simulink model "Final_Simulink_Model_assignment_2"  (R2022b)
settings: Solver=FixedStepAuto  StartTime=0.0  StopTime=inf  FixedStep=1e-3  RelTol=1e-3  EnableMultiTasking=on
undefined symbols (not defined in the file): A0, A1, ATR_PULSE_WIDTH, ATR_PUSLE_WIDTH, D0, D1, D10, D11, D12, D13, D2, D3, D4, D5, D6, D7, D8, D9, LRL, magnitude, PTA0, PTA1, PTA2, PTB2, PTB23, PTB3, PTB9, PTC16, PTC17, PTC2, PTC3, PTC4, PTD0, PTD1, PTD2, PTD3, REF_PERIOD, REF_PREIOD, VENT_PULSE_WIDTH
libraries: frdmk64flib x30, etargetslib x9, dspstat3 x1
(part 1 of 2)
settings Model: ExtModeTrigDuration=5  Creator=clara  LastModifiedBy=dinghao
settings OptimizationCC: EnhancedBackFolding=on  PassReuseOutputArgsAs=Individual arguments  ZeroExternalMemoryAtStartup=off  ZeroInternalMemoryAtStartup=off  MaxStackSize=64  OptimizeBlockOrder=speed  DifferentSizesBufferReuse=on  OptimizationCustomize=off  EfficientTunableParamExpr=on
settings DebuggingCC: ParameterTunabilityLossMsg=error
settings HardwareCC: ProdBitPerPointer=32  ProdBitPerSizeT=32  ProdBitPerPtrDiffT=32  ProdLargestAtomicInteger=Long  ProdLargestAtomicFloat=Double  ProdWordSize=32  ProdHWDeviceType=ARM Compatible->ARM Cortex
settings ModelReferenceCC: EnableRefExpFcnMdlSchedulingChecks=on
settings SFSimCC: MATLABDynamicMemAlloc=off
settings RTWCC: Description=Embedded Coder  SystemTargetFile=ert.tlc  HardwareBoard=NXP FRDM-K64F  TLCOptions="-aInlineSetEventsForThisBaseRateFcn=TLC_FALSE -aSuppressMultiTaskScheduler=TLC_FALSE  -aRateBasedStepFcn=0"  TemplateMakefile=ert_default_tmf  Toolchain=GNU Tools for ARM Embedded Processors
settings CodeAppCC: ForceParamTrailComments=on  IgnoreCustomStorageClasses=off  OperatorAnnotations=on  SimulinkDataObjDesc=on  SFDataObjDesc=on  InsertBlockDesc=on
settings ERTTargetCC: ExtModeTransport=4  ExtModeMexFile=sendToCommService

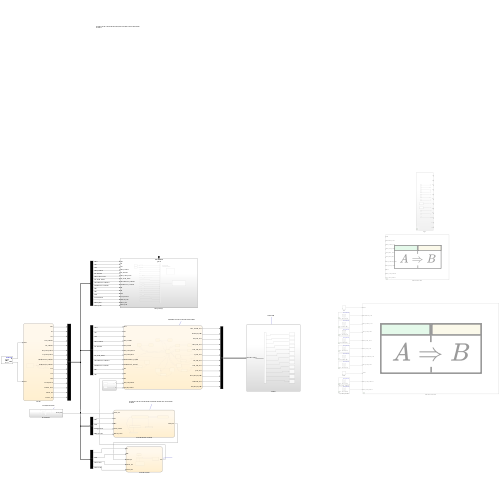
[thumbnail: Simulink's stored preview of the top-level diagram]
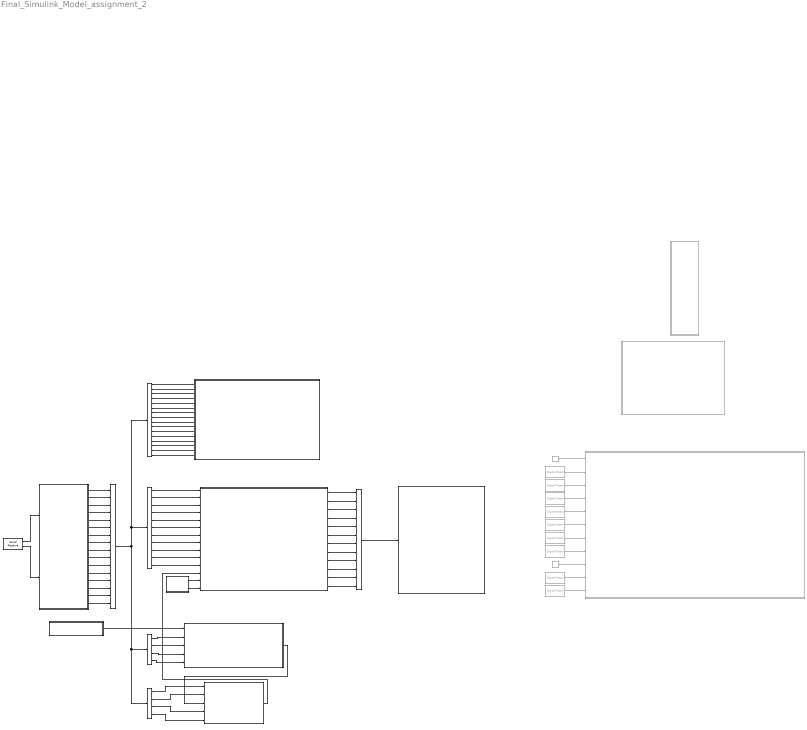
== system Final_Simulink_Model_assignment_2 ==
  note: the model is used to find the desired pacing rate with response factor under different conditions
  note: Find target activity level
  note: Slowly or linearly increase the current heart rate to the desired value
  note: the model is used to find the desired pacing rate with response factor under different conditions
  note: Output hiding
  note: Eight different modes with and without rate adaptive
  ATR_CMP_DETECT : frdmk64flib/Digital Read  Commented=on  Whichpin=PTC16 (D0)  SampleTime=-1
  Accelerometer1 : Subsystem
  Bus Creator : BusCreator  Inputs=16
  Bus Creator1 : BusCreator  Inputs=12
  Bus Selector : BusSelector  OutputSignals=mode,LRL,URL,VENT_Amplitude,ATR_Amplitude,VENT_PULSE_WIDTH,ATR_PULSE_WIDTH,VENTSENSITIVITY_Amplitude,ATRSENSITIVITY_Amplitude,ARP,VRP
  Bus Selector1 : BusSelector  OutputSignals=mode,LRL,URL,VENT_Amplitude,ATR_Amplitude,VENT_PULSE_WIDTH,ATR_PULSE_WIDTH,VENTSENSITIVITY_Amplitude,ATRSENSITIVITY_Amplitude,ARP,VRP,MSR,Activity_threshold,Response_Factor,Reaction_time,Recovery_time
  Bus Selector2 : BusSelector  OutputSignals=LRL,MSR,Activity_threshold,Response_Factor
  Bus Selector3 : BusSelector  OutputSignals=LRL,MSR,Reaction_time,Recovery_time
  COM_IN1 : Stateflow chart  TreatAsAtomicUnit=on
  Chart1 : Stateflow chart  TreatAsAtomicUnit=on
      settings: PortSchema="{\"entries\":[{\"content\":{\"sides\":[{\"content\":{\"connectorIds\":[\"In8\",\"In1\",\"In6\",\"In2\",\"In3\",\"In4\",\"In5\",\"In7\",\"In9\",\"In10\",\"In11\",\"In12\",\"In13\",\"In14\"]},\"type\":\"ConnectorPlacement.EquallySpacedRectSide\",\"uuid\":\"411cfc43-89c3-4653-9fab-0da98be593d3\"},{\"content\":{\"connectorIds\":[\"Out1\",\"Out2\",\"Out3\",\"Out4\",\"Out5\",\"Out6\",\"Out7\",\"Out8\",\"Out9\",\"Out10\",\"Out11\",\"Out12\"],\"side\":\"RIGHT\"},\"type\":\"ConnectorPlacement.EquallySpacedRectSide\",\"uuid\":\"ad1683f7-26aa-4767-b656-f3b731cb8235\"},{\"content\":{\"connectorIds\":[],\"side\":\"TOP\"},\"type\":\"ConnectorPlacement.EquallySpacedRectSide\",\"uuid\":\"fbccba07-c1cc-4c9f-8e56-0bdfb6912bb8\"}]},\"type\":\"ConnectorPlacement.EquallySpacedConnector\",\"uuid\":\"0c618a7f-9484-4de3-a6ac-3c8308721375\"}],\"packageUris\":[\"http://schema.mathworks.com/mf0/Connector/R2020b\"],\"version\":\"1.0\"}"
  Digital Read : frdmk64flib/Digital Read  Commented=on  Whichpin=PTB9 (D2)  SampleTime=-1
  Digital Read1 : frdmk64flib/Digital Read  Commented=on  Whichpin=PTD0 (D10)  SampleTime=-1
  Digital Read2 : frdmk64flib/Digital Read  Commented=on  Whichpin=PTD2 (D11)  SampleTime=-1
  Digital Read3 : frdmk64flib/Digital Read  Commented=on  Whichpin=PTA0 (D8)  SampleTime=-1
  Digital Read4 : frdmk64flib/Digital Read  Commented=on  Whichpin=PTD3 (D12)  SampleTime=-1
  Digital Read5 : frdmk64flib/Digital Read  Commented=on  Whichpin=PTC4 (D9)  SampleTime=-1
  Digital Read6 : frdmk64flib/Digital Read  Commented=on  Whichpin=PTD1 (D13)  SampleTime=-1
  Find the desired rate for pacing1 : Stateflow chart  TreatAsAtomicUnit=on
  Find the pacing rate1 : Stateflow chart  TreatAsAtomicUnit=on
  INPUT 1 : Subsystem  Commented=on
  Mode : Constant  Commented=on
  OUTPUT1 : Subsystem
  Requirements Table : Requirements Table  Commented=on  TreatAsAtomicUnit=on
  Requirements Table1 : Requirements Table  Commented=on  TreatAsAtomicUnit=on
  Serial Receive1 : frdmk64flib/Serial Receive  SCIModule=0  Baudrate=uint32(9600)  Parity=None  StopBits=1  HardwareFlowControl=None  ByteOrder=LittleEndian  DataType=uint8  DataLength=35  BlockingMode=off  OutputStatus=on  SampleTime=-1
  State : Constant  Commented=on
  Subsystem1 : Subsystem
  VENT_CMP_DETECT : frdmk64flib/Digital Read  Commented=on  Whichpin=PTC17 (D1)  SampleTime=-1
  send_params()1 : Subsystem
  wires:
  Accelerometer1/1(Activity_level) -> Find the desired rate for pacing1/1(Activity_level)
  Subsystem1/2(Out8) -> Chart1/14(ATR_CMP_DETECT)
  Serial Receive1/2 -> COM_IN1/2(status)
  Subsystem1/1(Out7) -> Chart1/13(VENT_CMP_DETECT)
  Find the pacing rate1/1(rate) -> Chart1/12(Rate)
  Find the desired rate for pacing1/1(Desired_rate) -> Find the pacing rate1/3(Desired_rate)
  Serial Receive1/1 -> COM_IN1/1(rxdata)
  COM_IN1/1(mode) -> Bus Creator/1
  COM_IN1/2(LRL) -> Bus Creator/2
  COM_IN1/3(URL) -> Bus Creator/3
  COM_IN1/4(VENT_Amplitude) -> Bus Creator/4
  COM_IN1/5(ATR_Amplitude) -> Bus Creator/5
  COM_IN1/6(VENT_PULSE_WIDTH) -> Bus Creator/6
  COM_IN1/7(ATR_PULSE_WIDTH) -> Bus Creator/7
  COM_IN1/8(VENTSENSITIVITY_Amplitude) -> Bus Creator/8
  COM_IN1/9(ATRSENSITIVITY_Amplitude) -> Bus Creator/9
  COM_IN1/10(ARP) -> Bus Creator/10
  COM_IN1/11(VRP) -> Bus Creator/11
  COM_IN1/12(MSR) -> Bus Creator/12
  COM_IN1/13(Activity_threshold) -> Bus Creator/13
  COM_IN1/14(Response_Factor) -> Bus Creator/14
  COM_IN1/15(Reaction_time) -> Bus Creator/15
  COM_IN1/16(Recovery_time) -> Bus Creator/16
  Bus Creator/1 -> Bus Selector3/1, Bus Selector2/1, Bus Selector1/1, Bus Selector/1
  Bus Selector/1 -> Chart1/8(mode)  "<mode>"
  Bus Selector/4 -> Chart1/2(VENT_Amplitude)  "<VENT_Amplitude>"
  Bus Selector/5 -> Chart1/3(ATR_Amplitude)  "<ATR_Amplitude>"
  Bus Selector/6 -> Chart1/4(VENT_PULSE_WIDTH)  "<VENT_PULSE_WIDTH>"
  Bus Selector/7 -> Chart1/5(ATR_PULSE_WIDTH)  "<ATR_PULSE_WIDTH>"
  Bus Selector/8 -> Chart1/7(VENTSENSITIVITY_Amplitude)  "<VENTSENSITIVITY_Amplitude>"
  Bus Selector/9 -> Chart1/9(ATRSENSITIVITY_Amplitude)  "<ATRSENSITIVITY_Amplitude>"
  Bus Selector/10 -> Chart1/10(ARP)  "<ARP>"
  Bus Selector/11 -> Chart1/11(VRP)  "<VRP>"
  Bus Selector/2 -> Chart1/1(LRL)  "<LRL>"
  Bus Selector/3 -> Chart1/6(URL)  "<URL>"
  Bus Selector1/1 -> send_params()1/1(mode)  "<mode>"
  Bus Selector1/2 -> send_params()1/2(LRL)  "<LRL>"
  Bus Selector1/3 -> send_params()1/3(URL)  "<URL>"
  Bus Selector1/4 -> send_params()1/4(VENT_Amplitude)  "<VENT_Amplitude>"
  Bus Selector1/5 -> send_params()1/5(ATR_Amplitude)  "<ATR_Amplitude>"
  Bus Selector1/6 -> send_params()1/6(VENT_PULSE_WIDTH)  "<VENT_PULSE_WIDTH>"
  Bus Selector1/7 -> send_params()1/7(ATR_PULSE_WIDTH)  "<ATR_PULSE_WIDTH>"
  Bus Selector1/8 -> send_params()1/8(VENTSENSITIVITY_Amplitude)  "<VENTSENSITIVITY_Amplitude>"
  Bus Selector1/9 -> send_params()1/9(ATRSENSITIVITY_Amplitude)  "<ATRSENSITIVITY_Amplitude>"
  Bus Selector1/10 -> send_params()1/10(ARP)  "<ARP>"
  Bus Selector1/11 -> send_params()1/11(VRP)  "<VRP>"
  Bus Selector1/12 -> send_params()1/12(MSR)  "<MSR>"
  Bus Selector1/13 -> send_params()1/13(Activity_threshold)  "<Activity_threshold>"
  Bus Selector1/14 -> send_params()1/14(Response_Factor)  "<Response_Factor>"
  Bus Selector1/15 -> send_params()1/15(Reaction_time)  "<Reaction_time>"
  Bus Selector1/16 -> send_params()1/16(Recovery_time)  "<Recovery_time>"
  Bus Selector2/1 -> Find the desired rate for pacing1/2(LRL)  "<LRL>"
  Bus Selector2/2 -> Find the desired rate for pacing1/3(MSR)  "<MSR>"
  Bus Selector2/3 -> Find the desired rate for pacing1/4(Activity_threshold)  "<Activity_threshold>"
  Bus Selector2/4 -> Find the desired rate for pacing1/5(Response_Factor)  "<Response_Factor>"
  Bus Selector3/1 -> Find the pacing rate1/1(LRL)  "<LRL>"
  Bus Selector3/2 -> Find the pacing rate1/2(MSR)  "<MSR>"
  Bus Selector3/3 -> Find the pacing rate1/4(Reaction_time)  "<Reaction_time>"
  Bus Selector3/4 -> Find the pacing rate1/5(Recovery_time)  "<Recovery_time>"
  Chart1/1(PACE_CHARGE_CTRL) -> Bus Creator1/1
  Chart1/2(PACING_REF_PWM) -> Bus Creator1/2
  Chart1/3(ATR_PACE_CTRL) -> Bus Creator1/3
  Chart1/4(VENT_PACE_CTRL) -> Bus Creator1/4
  Chart1/5(PACE_GND_CTRL) -> Bus Creator1/5
  Chart1/6(Z_VENT_CTRL) -> Bus Creator1/6
  Chart1/7(ATR_GND_CTRL) -> Bus Creator1/7
  Chart1/8(VENT_GND_CTRL) -> Bus Creator1/8
  Chart1/9(Z_ATR_CTRL) -> Bus Creator1/9
  Chart1/10(VENT_CMP_REF_PWM) -> Bus Creator1/10
  Chart1/11(FRONTEND_CTRL) -> Bus Creator1/11
  Chart1/12(ATR_CMP_REF_PWM) -> Bus Creator1/12
  Bus Creator1/1 -> OUTPUT1/1(CONTROL OUTPUT)
  State/1 -> Requirements Table1/1(State)
  Digital Read/1 -> Requirements Table1/7(PACE_CHARGE_CTRL)
  Digital Read2/1 -> Requirements Table1/6(ATR_GND_CTRL)
  Digital Read5/1 -> Requirements Table1/3(VENT_PACE_CTRL)
  Digital Read6/1 -> Requirements Table1/2(FRONTEND_CTRL)
  ATR_CMP_DETECT/1 -> Requirements Table1/11(ATR_CMP_DETECT)
  Digital Read4/1 -> Requirements Table1/4(VENT_GND_CTRL)
  VENT_CMP_DETECT/1 -> Requirements Table1/10(VENT_CMP_DETECT)
  Digital Read3/1 -> Requirements Table1/5(ATR_PACE_CTRL)
  Mode/1 -> Requirements Table1/9(Mode)
  Digital Read1/1 -> Requirements Table1/8(PACE_GND_CTRL)

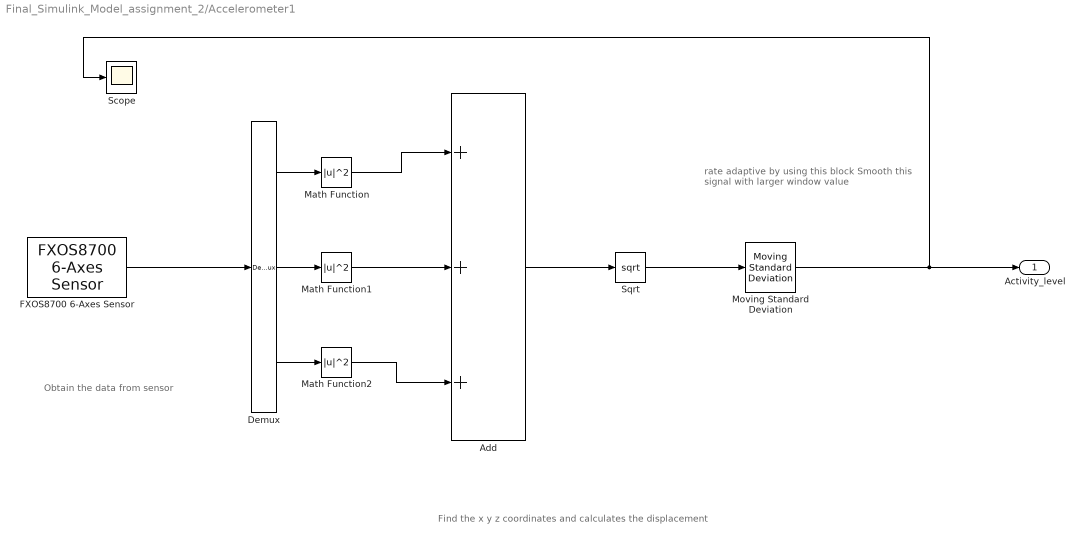
== system Final_Simulink_Model_assignment_2/Accelerometer1 ==
  note: Obtain the data from sensor
  note: Find the x y z coordinates and calculates the displacement
  note: rate adaptive by using this block
      | Smooth this signal with larger window value
  Add : Sum  Inputs=+++  OutDataTypeStr=double
  Demux : Demux  Outputs=3
  FXOS8700 6-Axes Sensor : frdmk64flib/FXOS8700 6-Axes Sensor  Activesensor=Accelerometer only  ODR=800Hz  HybridODR=400Hz  Accelfullrange=-4g to +4g  SampleTime=0.01
  Math Function : Math  Operator=magnitude^2  OutDataTypeStr=double
  Math Function1 : Math  Operator=magnitude^2  OutDataTypeStr=double
  Math Function2 : Math  Operator=magnitude^2  OutDataTypeStr=double
  Moving Standard Deviation : dspstat3/Moving Standard Deviation  Method=Sliding window  ForgettingFactorPort=off  SpecifyWindowLength=on  WindowLength=400  OverlapLength=399  AllowArbitraryInputLength=off  ForgettingFactor=0.9  SimulateUsing=Code generation
  Scope : Scope
  Sqrt : Sqrt  OutDataTypeStr=double
  Activity_level : Outport  OutDataTypeStr=double
  wires:
  FXOS8700 6-Axes Sensor/1 -> Demux/1
  Demux/1 -> Math Function/1
  Demux/2 -> Math Function1/1
  Demux/3 -> Math Function2/1
  Math Function/1 -> Add/1
  Math Function2/1 -> Add/3
  Math Function1/1 -> Add/2
  Add/1 -> Sqrt/1
  Sqrt/1 -> Moving Standard Deviation/1
  Moving Standard Deviation/1 -> Scope/1, Activity_level/1

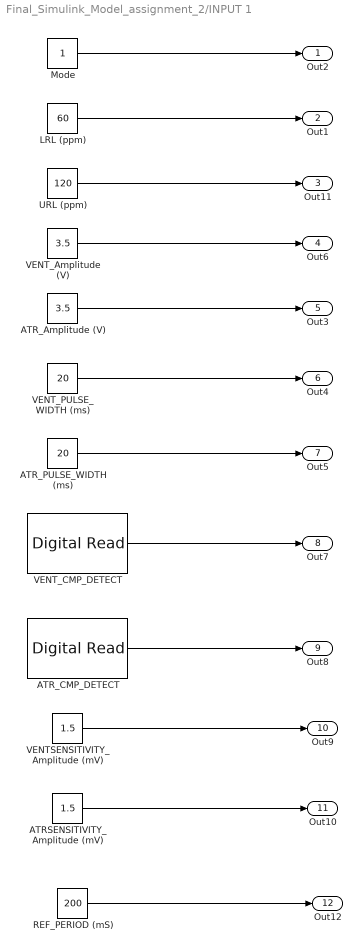
== system Final_Simulink_Model_assignment_2/INPUT 1 ==
  ATRSENSITIVITY_Amplitude (mV) : Constant  Value=1.5
  ATR_Amplitude (V) : Constant  Value=3.5
  ATR_CMP_DETECT : frdmk64flib/Digital Read  Whichpin=PTC16 (D0)  SampleTime=-1
  ATR_PULSE_WIDTH (ms) : Constant  Value=20
  LRL (ppm) : Constant  Value=60
  Mode : Constant
  REF_PERIOD (mS) : Constant  Value=200
  URL (ppm) : Constant  Value=120
  VENTSENSITIVITY_Amplitude (mV) : Constant  Value=1.5
  VENT_Amplitude (V) : Constant  Value=3.5
  VENT_CMP_DETECT : frdmk64flib/Digital Read  Whichpin=PTC17 (D1)  SampleTime=-1
  VENT_PULSE_WIDTH (ms) : Constant  Value=20
  Out2 : Outport
  Out1 : Outport  Port=2
  Out11 : Outport  Port=3
  Out6 : Outport  Port=4
  Out3 : Outport  Port=5
  Out4 : Outport  Port=6
  Out5 : Outport  Port=7
  Out7 : Outport  Port=8
  Out8 : Outport  Port=9
  Out9 : Outport  Port=10
  Out10 : Outport  Port=11
  Out12 : Outport  Port=12
  wires:
  LRL (ppm)/1 -> Out1/1
  VENT_PULSE_WIDTH (ms)/1 -> Out4/1
  VENT_Amplitude (V)/1 -> Out6/1
  URL (ppm)/1 -> Out11/1
  Mode/1 -> Out2/1
  ATR_Amplitude (V)/1 -> Out3/1
  ATR_PULSE_WIDTH (ms)/1 -> Out5/1
  VENT_CMP_DETECT/1 -> Out7/1
  ATR_CMP_DETECT/1 -> Out8/1
  VENTSENSITIVITY_Amplitude (mV)/1 -> Out9/1
  ATRSENSITIVITY_Amplitude (mV)/1 -> Out10/1
  REF_PERIOD (mS)/1 -> Out12/1

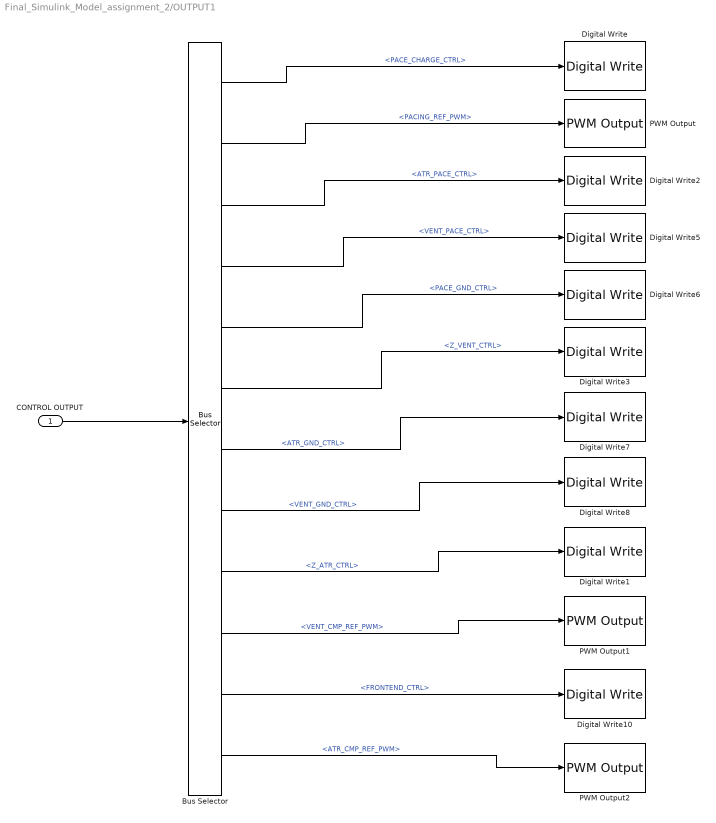
== system Final_Simulink_Model_assignment_2/OUTPUT1 ==
  CONTROL OUTPUT : Inport
  Bus Selector : BusSelector  OutputSignals=PACE_CHARGE_CTRL,PACING_REF_PWM,ATR_PACE_CTRL,VENT_PACE_CTRL,PACE_GND_CTRL,Z_VENT_CTRL,ATR_GND_CTRL,VENT_GND_CTRL,Z_ATR_CTRL,VENT_CMP_REF_PWM,FRONTEND_CTRL,ATR_CMP_REF_PWM
  Digital Write : frdmk64flib/Digital Write  Whichpin=PTB9 (D2)
  Digital Write1 : frdmk64flib/Digital Write  Whichpin=PTB23 (D4)
  Digital Write10 : frdmk64flib/Digital Write  Whichpin=PTD1 (D13)
  Digital Write2 : frdmk64flib/Digital Write  Whichpin=PTA0 (D8)
  Digital Write3 : frdmk64flib/Digital Write  Whichpin=PTC3 (D7)
  Digital Write5 : frdmk64flib/Digital Write  Whichpin=PTC4 (D9)
  Digital Write6 : frdmk64flib/Digital Write  Whichpin=PTD0 (D10)
  Digital Write7 : frdmk64flib/Digital Write  Whichpin=PTD2 (D11)
  Digital Write8 : frdmk64flib/Digital Write  Whichpin=PTD3 (D12)
  PWM Output : frdmk64flib/PWM Output  Whichpin=PTA2 (D5)  InitialFrequency=2000  InitialDutyCycle=0
  PWM Output1 : frdmk64flib/PWM Output  Whichpin=PTA1 (D3)  InitialFrequency=2000  InitialDutyCycle=0
  PWM Output2 : frdmk64flib/PWM Output  Whichpin=PTC2 (D6)  InitialFrequency=2000  InitialDutyCycle=0
  wires:
  CONTROL OUTPUT/1 -> Bus Selector/1
  Bus Selector/1 -> Digital Write/1  "<PACE_CHARGE_CTRL>"
  Bus Selector/2 -> PWM Output/1  "<PACING_REF_PWM>"
  Bus Selector/3 -> Digital Write2/1  "<ATR_PACE_CTRL>"
  Bus Selector/4 -> Digital Write5/1  "<VENT_PACE_CTRL>"
  Bus Selector/5 -> Digital Write6/1  "<PACE_GND_CTRL>"
  Bus Selector/6 -> Digital Write3/1  "<Z_VENT_CTRL>"
  Bus Selector/7 -> Digital Write7/1  "<ATR_GND_CTRL>"
  Bus Selector/8 -> Digital Write8/1  "<VENT_GND_CTRL>"
  Bus Selector/9 -> Digital Write1/1  "<Z_ATR_CTRL>"
  Bus Selector/10 -> PWM Output1/1  "<VENT_CMP_REF_PWM>"
  Bus Selector/11 -> Digital Write10/1  "<FRONTEND_CTRL>"
  Bus Selector/12 -> PWM Output2/1  "<ATR_CMP_REF_PWM>"

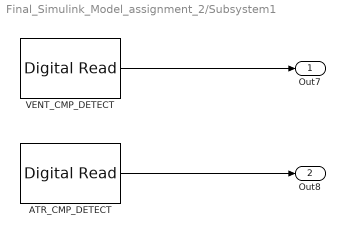
== system Final_Simulink_Model_assignment_2/Subsystem1 ==
  ATR_CMP_DETECT : frdmk64flib/Digital Read  Whichpin=PTC16 (D0)  SampleTime=-1
  VENT_CMP_DETECT : frdmk64flib/Digital Read  Whichpin=PTC17 (D1)  SampleTime=-1
  Out7 : Outport
  Out8 : Outport  Port=2
  wires:
  ATR_CMP_DETECT/1 -> Out8/1
  VENT_CMP_DETECT/1 -> Out7/1

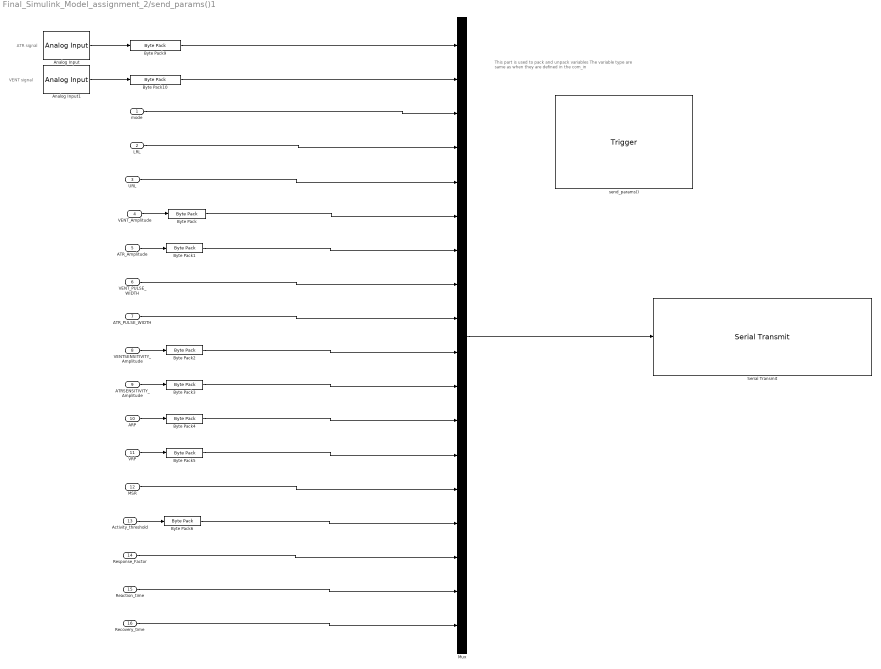
== system Final_Simulink_Model_assignment_2/send_params()1 ==
  note: This part is used to pack and unpack variables
      | The variable type are same as when they are defined in the com_in
  note: ATR signal
  note: VENT signal
  mode : Inport
  LRL : Inport  Port=2
  URL : Inport  Port=3
  VENT_Amplitude : Inport  Port=4
  ATR_Amplitude : Inport  Port=5
  VENT_PULSE_WIDTH : Inport  Port=6
  ATR_PULSE_WIDTH : Inport  Port=7
  VENTSENSITIVITY_Amplitude : Inport  Port=8
  ATRSENSITIVITY_Amplitude : Inport  Port=9
  ARP : Inport  Port=10
  VRP : Inport  Port=11
  MSR : Inport  Port=12
  Activity_threshold : Inport  Port=13
  Response_Factor : Inport  Port=14
  Reaction_time : Inport  Port=15
  Recovery_time : Inport  Port=16
  send_params() : TriggerPort  TriggerType=function-call  IsSimulinkFunction=on  FunctionName=send_params  VariantControl=Variant
  Analog Input : frdmk64flib/Analog Input  Whichpin=PTB2 (A0)  SampleTime=-1
  Analog Input1 : frdmk64flib/Analog Input  Whichpin=PTB3 (A1)  SampleTime=-1
  Byte Pack{,1..3,6} (5 alike) : etargetslib/Byte Pack  datatypes={'single'}  byteAlign=1
  Byte Pack10 : etargetslib/Byte Pack  datatypes={'double'}  byteAlign=1
  Byte Pack4 : etargetslib/Byte Pack  datatypes={'uint16'}  byteAlign=1
  Byte Pack5 : etargetslib/Byte Pack  datatypes={'uint16'}  byteAlign=1
  Byte Pack9 : etargetslib/Byte Pack  datatypes={'double'}  byteAlign=1
  Mux : Mux  Inputs=18
  Serial Transmit : frdmk64flib/Serial Transmit  SCIModule=0  Baudrate=uint32(9600)  Parity=None  StopBits=1  HardwareFlowControl=None  ByteOrder=LittleEndian  BlockingMode=on  OutputStatus=off
  wires:
  mode/1 -> Mux/3
  LRL/1 -> Mux/4
  URL/1 -> Mux/5
  VENT_Amplitude/1 -> Byte Pack/1
  Byte Pack/1 -> Mux/6
  ATR_Amplitude/1 -> Byte Pack1/1
  Byte Pack1/1 -> Mux/7
  VENT_PULSE_WIDTH/1 -> Mux/8
  ATR_PULSE_WIDTH/1 -> Mux/9
  VENTSENSITIVITY_Amplitude/1 -> Byte Pack2/1
  Byte Pack2/1 -> Mux/10
  ATRSENSITIVITY_Amplitude/1 -> Byte Pack3/1
  Byte Pack3/1 -> Mux/11
  Byte Pack4/1 -> Mux/12
  ARP/1 -> Byte Pack4/1
  VRP/1 -> Byte Pack5/1
  Byte Pack5/1 -> Mux/13
  MSR/1 -> Mux/14
  Activity_threshold/1 -> Byte Pack6/1
  Byte Pack6/1 -> Mux/15
  Response_Factor/1 -> Mux/16
  Reaction_time/1 -> Mux/17
  Recovery_time/1 -> Mux/18
  Mux/1 -> Serial Transmit/1
  Analog Input/1 -> Byte Pack9/1
  Analog Input1/1 -> Byte Pack10/1
  Byte Pack9/1 -> Mux/1
  Byte Pack10/1 -> Mux/2

== stateflow chart Final_Simulink_Model_assignment_2/Requirements Table ==
  (default) -> (junction 1073743363)
  (junction 1073743363) -> (junction 1073743364) : {
      | % SF_REQ_REV_07
      | }
  (junction 1073743364) -> (junction 1073743366) : {
      | % HEADER_ASSIGNMENTS
      |
      | }
  (junction 1073743366) -> (junction 1073743368) : {
      | % START_A_4
      | }
  (junction 1073743368) -> (junction 1073743370) : {
      | }
  (junction 1073743370) -> (junction 1073743372)
  (junction 1073743372) -> (junction 1073743374) : {
      | }
  (junction 1073743374) -> (junction 1073743376) : {
      | % END_A_4
      | }
  (junction 1073743376) -> (junction 1073743378) : {
      | % START_R_1
      | }
  (junction 1073743378) -> (junction 1073743380) : {
      | }
  (junction 1073743380) -> (junction 1073743382)
  (junction 1073743382) -> (junction 1073743384) [order 1] : [(((Mode) == (1)))]
  (junction 1073743382) -> (junction 1073743426) [order 2]
  (junction 1073743384) -> (junction 1073743386) : {
      |
      |
      | }
  (junction 1073743386) -> (junction 1073743388) : {
      | }
  (junction 1073743388) -> (junction 1073743390) : {
      | % START_R_7
      | }
  (junction 1073743390) -> (junction 1073743392) : {
      | }
  (junction 1073743392) -> (junction 1073743394)
  (junction 1073743394) -> (junction 1073743396) [order 1] : [duration((((State) == (1)))) >= 60000/LRL - ATR_PUSLE_WIDTH]
  (junction 1073743394) -> (junction 1073743402) [order 2]
  (junction 1073743396) -> (junction 1073743398) : {
      | reqtable_postcondition((((ATR_PACE_CTRL) == (1))) && (((ATR_GND_CTRL) == (0))) && (((PACE_CHARGE_CTRL) == (0))) && (((PACE_GND_CTRL) == (1))), 'R:1.1');
      |
      |
      | }
  (junction 1073743398) -> (junction 1073743400) : {
      | }
  (junction 1073743400) -> (junction 1073743402)
  (junction 1073743402) -> (junction 1073743404)
  (junction 1073743404) -> (junction 1073743406) : {
      | % END_R_7
      | }
  (junction 1073743406) -> (junction 1073743408) : {
      | % START_R_10
      | }
  (junction 1073743408) -> (junction 1073743410) : {
      | }
  (junction 1073743410) -> (junction 1073743412)
  (junction 1073743412) -> (junction 1073743414) [order 1] : [duration((((State) == (2)))) >= ATR_PULSE_WIDTH]
  (junction 1073743412) -> (junction 1073743420) [order 2]
  (junction 1073743414) -> (junction 1073743416) : {
      | reqtable_postcondition((((ATR_PACE_CTRL) == (0))) && (((ATR_GND_CTRL) == (1))) && (((PACE_CHARGE_CTRL) == (1))) && (((PACE_GND_CTRL) == (1))), 'R:1.2');
      |
      |
      | }
  (junction 1073743416) -> (junction 1073743418) : {
      | }
  (junction 1073743418) -> (junction 1073743420)
  (junction 1073743420) -> (junction 1073743422)
  (junction 1073743422) -> (junction 1073743424) : {
      | % END_R_10
      | }
  (junction 1073743424) -> (junction 1073743426)
  (junction 1073743426) -> (junction 1073743428)
  (junction 1073743428) -> (junction 1073743430) : {
      | % END_R_1
      | }
  (junction 1073743430) -> (junction 1073743432) : {
      | % START_R_13
      | }
  (junction 1073743432) -> (junction 1073743434) : {
      | }
  (junction 1073743434) -> (junction 1073743436)
  (junction 1073743436) -> (junction 1073743438) [order 1] : [(((Mode) == (2)))]
  (junction 1073743436) -> (junction 1073743480) [order 2]
  (junction 1073743438) -> (junction 1073743440) : {
      |
      |
      | }
  (junction 1073743440) -> (junction 1073743442) : {
      | }
  (junction 1073743442) -> (junction 1073743444) : {
      | % START_R_16
      | }
  (junction 1073743444) -> (junction 1073743446) : {
      | }
  (junction 1073743446) -> (junction 1073743448)
  (junction 1073743448) -> (junction 1073743450) [order 1] : [duration((((State) == (1)))) >= 60000/LRL - VENT_PULSE_WIDTH]
  (junction 1073743448) -> (junction 1073743456) [order 2]
  (junction 1073743450) -> (junction 1073743452) : {
      | reqtable_postcondition((((PACE_CHARGE_CTRL) == (0))) && (((PACE_GND_CTRL) == (1))) && (((VENT_PACE_CTRL) == (1))) && (((VENT_GND_CTRL) == (0))), 'R:2.1');
      |
      |
      | }
  (junction 1073743452) -> (junction 1073743454) : {
      | }
  (junction 1073743454) -> (junction 1073743456)
  (junction 1073743456) -> (junction 1073743458)
  (junction 1073743458) -> (junction 1073743460) : {
      | % END_R_16
      | }
  (junction 1073743460) -> (junction 1073743462) : {
      | % START_R_19
      | }
  (junction 1073743462) -> (junction 1073743464) : {
      | }
  (junction 1073743464) -> (junction 1073743466)
  (junction 1073743466) -> (junction 1073743468) [order 1] : [duration((((State) == (2)))) >= VENT_PULSE_WIDTH]
  (junction 1073743466) -> (junction 1073743474) [order 2]
  (junction 1073743468) -> (junction 1073743470) : {
      | reqtable_postcondition((((PACE_CHARGE_CTRL) == (1))) && (((PACE_GND_CTRL) == (1))) && (((VENT_PACE_CTRL) == (0))) && (((VENT_GND_CTRL) == (1))), 'R:2.2');
      |
      |
      | }
  (junction 1073743470) -> (junction 1073743472) : {
      | }
  (junction 1073743472) -> (junction 1073743474)
  (junction 1073743474) -> (junction 1073743476)
  (junction 1073743476) -> (junction 1073743478) : {
      | % END_R_19
      | }
  (junction 1073743478) -> (junction 1073743480)
  (junction 1073743480) -> (junction 1073743482)
  (junction 1073743482) -> (junction 1073743484) : {
      | % END_R_13
      | }
  (junction 1073743484) -> (junction 1073743486) : {
      | % START_R_22
      | }
  (junction 1073743486) -> (junction 1073743488) : {
      | }
  (junction 1073743488) -> (junction 1073743490)
  (junction 1073743490) -> (junction 1073743492) [order 1] : [(((Mode) == (3)))]
  (junction 1073743490) -> (junction 1073743552) [order 2]
  (junction 1073743492) -> (junction 1073743494) : {
      |
      |
      | }
  (junction 1073743494) -> (junction 1073743496) : {
      | }
  (junction 1073743496) -> (junction 1073743498) : {
      | % START_R_25
      | }
  (junction 1073743498) -> (junction 1073743500) : {
      | }
  (junction 1073743500) -> (junction 1073743502)
  (junction 1073743502) -> (junction 1073743504) [order 1] : [duration((((State) == (1)))) >= 60000/LRL - ATR_PULSE_WIDTH]
  (junction 1073743502) -> (junction 1073743510) [order 2]
  (junction 1073743504) -> (junction 1073743506) : {
      | reqtable_postcondition((((ATR_PACE_CTRL) == (0))) && (((ATR_GND_CTRL) == (1))) && (((PACE_CHARGE_CTRL) == (1))) && (((PACE_GND_CTRL) == (1))) && (((FRONTEND_CTRL) == (1))), 'R:3.1');
      |
      |
      | }
  (junction 1073743506) -> (junction 1073743508) : {
      | }
  (junction 1073743508) -> (junction 1073743510)
  (junction 1073743510) -> (junction 1073743512)
  (junction 1073743512) -> (junction 1073743514) : {
      | % END_R_25
      | }
  (junction 1073743514) -> (junction 1073743516) : {
      | % START_R_28
      | }
  (junction 1073743516) -> (junction 1073743518) : {
      | }
  (junction 1073743518) -> (junction 1073743520)
  (junction 1073743520) -> (junction 1073743522) [order 1] : [duration((((State) == (2)))) >= ATR_PULSE_WIDTH]
  (junction 1073743520) -> (junction 1073743528) [order 2]
  (junction 1073743522) -> (junction 1073743524) : {
      | reqtable_postcondition((((ATR_PACE_CTRL) == (1))) && (((ATR_GND_CTRL) == (0))) && (((PACE_CHARGE_CTRL) == (0))) && (((PACE_GND_CTRL) == (1))), 'R:3.2');
      |
      |
      | }
  (junction 1073743524) -> (junction 1073743526) : {
      | }
  (junction 1073743526) -> (junction 1073743528)
  (junction 1073743528) -> (junction 1073743530)
  (junction 1073743530) -> (junction 1073743532) : {
      | % END_R_28
      | }
  (junction 1073743532) -> (junction 1073743534) : {
      | % START_R_31
      | }
  (junction 1073743534) -> (junction 1073743536) : {
      | }
  (junction 1073743536) -> (junction 1073743538)
  (junction 1073743538) -> (junction 1073743540) [order 1] : [duration((((State) == (3)))) >= REF_PERIOD]
  (junction 1073743538) -> (junction 1073743546) [order 2]
  (junction 1073743540) -> (junction 1073743542) : {
      | reqtable_postcondition((((ATR_PACE_CTRL) == (0))) && (((ATR_GND_CTRL) == (1))) && (((PACE_CHARGE_CTRL) == (0))) && (((PACE_GND_CTRL) == (1))) && (((FRONTEND_CTRL) == (0))), 'R:3.3');
      |
      |
      | }
  (junction 1073743542) -> (junction 1073743544) : {
      | }
  (junction 1073743544) -> (junction 1073743546)
  (junction 1073743546) -> (junction 1073743548)
  (junction 1073743548) -> (junction 1073743550) : {
      | % END_R_31
      | }
  (junction 1073743550) -> (junction 1073743552)
  (junction 1073743552) -> (junction 1073743554)
  (junction 1073743554) -> (junction 1073743556) : {
      | % END_R_22
      | }
  (junction 1073743556) -> (junction 1073743558) : {
      | % START_R_34
      | }
  (junction 1073743558) -> (junction 1073743560) : {
      | }
  (junction 1073743560) -> (junction 1073743562)
  (junction 1073743562) -> (junction 1073743564) [order 1] : [(((Mode) == (4)))]
  (junction 1073743562) -> (junction 1073743624) [order 2]
  (junction 1073743564) -> (junction 1073743566) : {
      |
      |
      | }
  (junction 1073743566) -> (junction 1073743568) : {
      | }
  (junction 1073743568) -> (junction 1073743570) : {
      | % START_R_37
      | }
  (junction 1073743570) -> (junction 1073743572) : {
      | }
  (junction 1073743572) -> (junction 1073743574)
  (junction 1073743574) -> (junction 1073743576) [order 1] : [duration((((State) == (1)))) >= 60000/LRL - VENT_PULSE_WIDTH]
  (junction 1073743574) -> (junction 1073743582) [order 2]
  (junction 1073743576) -> (junction 1073743578) : {
      | reqtable_postcondition((((PACE_CHARGE_CTRL) == (1))) && (((PACE_GND_CTRL) == (1))) && (((VENT_PACE_CTRL) == (0))) && (((VENT_GND_CTRL) == (1))) && (((FRONTEND_CTRL) == (1))), 'R:4.1');
      |
      |
      | }
  (junction 1073743578) -> (junction 1073743580) : {
      | }
  (junction 1073743580) -> (junction 1073743582)
  (junction 1073743582) -> (junction 1073743584)
  (junction 1073743584) -> (junction 1073743586) : {
      | % END_R_37
      | }
  (junction 1073743586) -> (junction 1073743588) : {
      | % START_R_40
      | }
  (junction 1073743588) -> (junction 1073743590) : {
      | }
  (junction 1073743590) -> (junction 1073743592)
  (junction 1073743592) -> (junction 1073743594) [order 1] : [duration((((State) == (2)))) >= VENT_PULSE_WIDTH]
  (junction 1073743592) -> (junction 1073743600) [order 2]
  (junction 1073743594) -> (junction 1073743596) : {
      | reqtable_postcondition((((PACE_CHARGE_CTRL) == (0))) && (((PACE_GND_CTRL) == (1))) && (((VENT_PACE_CTRL) == (1))) && (((VENT_GND_CTRL) == (0))), 'R:4.2');
      |
      |
      | }
  (junction 1073743596) -> (junction 1073743598) : {
      | }
  (junction 1073743598) -> (junction 1073743600)
  (junction 1073743600) -> (junction 1073743602)
  (junction 1073743602) -> (junction 1073743604) : {
      | % END_R_40
      | }
  (junction 1073743604) -> (junction 1073743606) : {
      | % START_R_43
      | }
  (junction 1073743606) -> (junction 1073743608) : {
      | }
  (junction 1073743608) -> (junction 1073743610)
  (junction 1073743610) -> (junction 1073743612) [order 1] : [duration((((State) == (3)))) >= REF_PREIOD]
  (junction 1073743610) -> (junction 1073743618) [order 2]
  (junction 1073743612) -> (junction 1073743614) : {
      | reqtable_postcondition((((PACE_CHARGE_CTRL) == (0))) && (((PACE_GND_CTRL) == (1))) && (((VENT_PACE_CTRL) == (0))) && (((VENT_GND_CTRL) == (1))) && (((FRONTEND_CTRL) == (0))), 'R:4.3');
      |
      |
      | }
  (junction 1073743614) -> (junction 1073743616) : {
      | }
  (junction 1073743616) -> (junction 1073743618)
  (junction 1073743618) -> (junction 1073743620)
  (junction 1073743620) -> (junction 1073743622) : {
      | % END_R_43
      | }
  (junction 1073743622) -> (junction 1073743624)
  (junction 1073743624) -> (junction 1073743626)
  (junction 1073743626) -> (junction 1073743628) : {
      | % END_R_34
      | }
  data: State input; FRONTEND_CTRL input; VENT_PACE_CTRL input; VENT_GND_CTRL input; ATR_PACE_CTRL input; ATR_GND_CTRL input; PACE_CHARGE_CTRL input; PACE_GND_CTRL input; Mode input double; VENT_CMP_DETECT input; ATR_CMP_DETECT input; ATR_PULSE_WIDTH parameter; LRL parameter; ATR_PUSLE_WIDTH parameter; VENT_PULSE_WIDTH parameter; REF_PREIOD parameter; REF_PERIOD parameter

== stateflow chart Final_Simulink_Model_assignment_2/COM_IN1 ==
  settings: executeAtInitialization=1
  note: Define a datatype and a size of each variable
  state SET_PARAM
    entry:
    mode = rxdata(3);
    LRL = rxdata(4);
    URL = rxdata(5);
    VENT_Amplitude = typecast(rxdata(6:9),'single');
    ATR_Amplitude = typecast(rxdata(10:13),'single');
    VENT_PULSE_WIDTH = rxdata(14);
    ATR_PULSE_WIDTH = rxdata(15);
    VENTSENSITIVITY_Amplitude = typecast(rxdata(16:19),'single');
    ATRSENSITIVITY_Amplitude = typecast(rxdata(20:23),'single');
    ARP = typecast(rxdata(24:25),'uint16');
    VRP = typecast(rxdata(26:27),'uint16');
    MSR = rxdata(28);
    Activity_threshold = typecast(rxdata(29:32),'single');
    Response_Factor = rxdata(33);
    Reaction_time = (rxdata(34));
    Recovery_time = (rxdata(35));
  note: Default value for every variable in this model.
  state Initialize
    entry:
    mode = 5; % 8 modes in total [1,8]
    LRL = 60; %ppm
    URL = 120; %ppm
    VENT_Amplitude = 3.5; %V
    ATR_Amplitude = 3.5; %V
    VENT_PULSE_WIDTH = 10; % ms
    ATR_PULSE_WIDTH = 10; % ms
    VENTSENSITIVITY_Amplitude = 1.5; %mV
    ATRSENSITIVITY_Amplitude = 1.5; %mV
    ARP = 250; %ms
    VRP = 250; %ms
    MSR = 120; % ppm maximum sensor rate
    Activity_threshold = 1.1; % output of accelerometer shell exceed this value
    Response_Factor = 8; % [1,16]
    Reaction_time = 30; % sec
    Recovery_time = 50; %sec
  state STANDBY
    %waiting for COM
  state ECHO_PARAM
    entry:
    send_params();
  SET_PARAM -> STANDBY
  (junction 15) -> SET_PARAM [order 1] : [rxdata(2) == hex2dec('55')]
  (default) -> Initialize
  STANDBY -> (junction 13) : [status == 0]
  (junction 13) -> (junction 15) [order 1] : [rxdata(1) == hex2dec('16')]
  (junction 13) -> STANDBY [order 2]
  (junction 15) -> ECHO_PARAM [order 2] : [rxdata(2) == hex2dec('22')]
  Initialize -> STANDBY
  ECHO_PARAM -> STANDBY
  data: rxdata input uint8; status input uint8; mode output uint8; LRL output uint8; URL output uint8; VENT_Amplitude output single; ATR_Amplitude output single; VENT_PULSE_WIDTH output uint8; ATR_PULSE_WIDTH output uint8; VENTSENSITIVITY_Amplitude output single; ATRSENSITIVITY_Amplitude output single; ARP output uint16; VRP output uint16; MSR output uint8; Activity_threshold output single; Response_Factor output uint8; Reaction_time output uint8; Recovery_time output uint8

== stateflow chart Final_Simulink_Model_assignment_2/Chart1 ==
  note: Pace ready
  state AOOR
    entry:
    % charge condition for C22
    ATR_PACE_CTRL = false;
    PACE_CHARGE_CTRL = true;
    % discharge condition for C21;
    ATR_GND_CTRL = true;
    PACE_GND_CTRL = true;
    %
    PACING_REF_PWM = 20*ATR_Amplitude;
  state Pacing_AOOR
    entry:
    PACE_CHARGE_CTRL = false;
    PACE_GND_CTRL = true;
    ATR_PACE_CTRL = true;
    ATR_GND_CTRL = false;
    %
  note: Recharge ready
  note: Pace ready
  state VOOR
    entry:
    % charge condition for C22
    VENT_PACE_CTRL = false;
    PACE_CHARGE_CTRL = true;
    % discharge condition for C21;
    VENT_GND_CTRL = true;
    PACE_GND_CTRL = true;
    %
    PACING_REF_PWM = 20*VENT_Amplitude;
  state Pacing_VOOR
    entry:
    PACE_CHARGE_CTRL = false;
    PACE_GND_CTRL = true;
    VENT_GND_CTRL = false;
    VENT_PACE_CTRL = true;
    %
  note: Pace ready
  state Pacing_AOO
    entry:
    PACE_CHARGE_CTRL = false;
    PACE_GND_CTRL = true;
    ATR_PACE_CTRL = true;
    ATR_GND_CTRL = false;
    %
  state AOO
    entry:
    % charge condition for C22
    ATR_PACE_CTRL = false;
    PACE_CHARGE_CTRL = true;
    % discharge condition for C21;
    ATR_GND_CTRL = true;
    PACE_GND_CTRL = true;
    %
    PACING_REF_PWM = 20*ATR_Amplitude;
  note: Recharge ready
  note: Charge C22 and discharge blocking capacitor
  note: Discharge C22 into atrium (charge C21)
  note: Pace ready
  state VOO
    entry:
    % charge condition for C22
    VENT_PACE_CTRL = false;
    PACE_CHARGE_CTRL = true;
    % discharge condition for C21;
    VENT_GND_CTRL = true;
    PACE_GND_CTRL = true;
    %
    PACING_REF_PWM = 20*VENT_Amplitude;
  state Pacing_VOO
    entry:
    PACE_CHARGE_CTRL = false;
    PACE_GND_CTRL = true;
    VENT_GND_CTRL = false;
    VENT_PACE_CTRL = true;
    %
  state MAIN
    entry:
    VENT_GND_CTRL=false;
    Z_ATR_CTRL = false;
    Z_VENT_CTRL = false;
    FRONTEND_CTRL=false;
    PACE_CHARGE_CTRL = false;
    VENT_PACE_CTRL = false;
    ATR_PACE_CTRL = false;
    PACE_GND_CTRL=false;
    ATR_GND_CTRL=false;
    note: Initial conditions
  note: Recharge ready
  note: Charge C22 and discharge blocking capacitor
  note: Discharge C22 into ventrical (charge C21)
  note: Begin sensing, charge C22 and discharge
      | blocking capacitor
  note: Discharge C22 into atrium (charge C21)
  note: If no signal is sensed
  state AAI
    entry:
    % begin sensing
    FRONTEND_CTRL = true;
    % charge condition for C22
    ATR_PACE_CTRL = false;
    PACE_CHARGE_CTRL = true;
    % discharge condition for C21;
    ATR_GND_CTRL = true;
    PACE_GND_CTRL = true;
    %
    PACING_REF_PWM = 20*ATR_Amplitude;
    ATR_CMP_REF_PWM = 20*ATRSENSITIVITY_Amplitude;
  state Pacing_AAI1
    entry:
    PACE_CHARGE_CTRL = false;
    PACE_GND_CTRL = true;
    ATR_PACE_CTRL = true;
    ATR_GND_CTRL = false;
    %
    PACING_REF_PWM = 20*ATR_Amplitude;
  note: If signal is sensed
  state AAI_REFRACTORY
    entry:
    FRONTEND_CTRL = false;
    ATR_PACE_CTRL = false;
    ATR_GND_CTRL = true;
    PACING_REF_PWM = 20*ATR_Amplitude;
    PACE_CHARGE_CTRL = false;
    PACE_GND_CTRL = true;
  note: If no signal is sensed
  note: If signal is sensed
  state Pacing_AAIR
    entry:
    PACE_CHARGE_CTRL = false;
    PACE_GND_CTRL = true;
    ATR_PACE_CTRL = true;
    ATR_GND_CTRL = false;
    %
    PACING_REF_PWM = 20*ATR_Amplitude;
  state AAIR
    entry:
    % begin sensing
    FRONTEND_CTRL = true;
    % charge condition for C22
    ATR_PACE_CTRL = false;
    PACE_CHARGE_CTRL = true;
    % discharge condition for C21;
    ATR_GND_CTRL = true;
    PACE_GND_CTRL = true;
    %
    PACING_REF_PWM = 20*ATR_Amplitude;
    ATR_CMP_REF_PWM = 20*ATRSENSITIVITY_Amplitude;
  note: Follows events during which senses
      | in the atrium are ignored
  note: Begin sensing, charge C22 and discharge
      | blocking capacitor
  note: Discharge C22 into ventrical (charge C21)
  note: If no signal is sensed
  note: If signal is sensed
  state Pacing_VVI
    entry:
    PACE_CHARGE_CTRL = false;
    PACE_GND_CTRL = true;
    VENT_GND_CTRL = false;
    VENT_PACE_CTRL = true;
    %
    PACING_REF_PWM = 20*VENT_Amplitude;
  state VVI
    entry:
    % begin sensing
    FRONTEND_CTRL = true;
    % charge condition for C22
    VENT_PACE_CTRL = false;
    PACE_CHARGE_CTRL = true;
    % discharge condition for C21;
    VENT_GND_CTRL = true;
    PACE_GND_CTRL = true;
    %
    PACING_REF_PWM = 20*VENT_Amplitude;
    VENT_CMP_REF_PWM = 20*VENTSENSITIVITY_Amplitude;
  state AAIR_REFRACTORY
    entry:
    FRONTEND_CTRL = false;
    ATR_PACE_CTRL = false;
    ATR_GND_CTRL = true;
    PACING_REF_PWM = 20*ATR_Amplitude;
    PACE_CHARGE_CTRL = false;
    PACE_GND_CTRL = true;
  note: If signal is sensed
  note: If signal is sensed
  note: Follows events during which senses
      | in the atrium are ignored
  note: If no signal is sensed
  state Pacing_VVIR
    entry:
    PACE_CHARGE_CTRL = false;
    PACE_GND_CTRL = true;
    VENT_GND_CTRL = false;
    VENT_PACE_CTRL = true;
    %
    PACING_REF_PWM = 20*VENT_Amplitude;
  state VVIR
    entry:
    % begin sensing
    FRONTEND_CTRL = true;
    % charge condition for C22
    VENT_PACE_CTRL = false;
    PACE_CHARGE_CTRL = true;
    % discharge condition for C21;
    VENT_GND_CTRL = true;
    PACE_GND_CTRL = true;
    %
    PACING_REF_PWM = 20*VENT_Amplitude;
    VENT_CMP_REF_PWM = 20*VENTSENSITIVITY_Amplitude;
  state VVI_REFRACTORY
    entry:
    FRONTEND_CTRL = false;
    VENT_GND_CTRL = true;
    PACING_REF_PWM = 20*VENT_Amplitude;
    PACE_CHARGE_CTRL = false;
    PACE_GND_CTRL = true;
  note: If signal is sensed
  note: If signal is sensed
  note: Follows events during which senses
      | in the ventrical are ignored
  state VVIR_REFRACTORY
    entry:
    FRONTEND_CTRL = false;
    VENT_GND_CTRL = true;
    PACING_REF_PWM = 20*VENT_Amplitude;
    PACE_CHARGE_CTRL = false;
    PACE_GND_CTRL = true;
  note: If signal is sensed
  AOOR -> Pacing_AOOR [order 1] : [after(60000/Rate - ATR_PULSE_WIDTH,msec)]
  Pacing_AOOR -> AOOR : [after(ATR_PULSE_WIDTH,msec)]
  AOOR -> MAIN [order 2] : [mode ~= 5]
  MAIN -> AOOR [order 5] : [mode == 5]
  VOOR -> Pacing_VOOR [order 1] : [after(60000/Rate - VENT_PULSE_WIDTH,msec)]
  AOO -> Pacing_AOO [order 1] : after((60000/LRL - ATR_PULSE_WIDTH),msec)
  MAIN -> AOO [order 4] : [mode == 1]
  Pacing_VOOR -> VOOR : [after(VENT_PULSE_WIDTH,msec)]
  Pacing_AOO -> AOO : [after(ATR_PULSE_WIDTH,msec)]
  MAIN -> VOOR [order 6] : [mode == 6]
  VOOR -> MAIN [order 2] : [mode ~= 6]
  AOO -> MAIN [order 2] : [mode ~= 1]
  MAIN -> VOO [order 1] : [mode == 2]
  (default) -> MAIN
  VOO -> Pacing_VOO [order 1] : [after(60000/LRL - VENT_PULSE_WIDTH,msec)]
  VOO -> MAIN [order 2] : [mode ~= 2]
  Pacing_VOO -> VOO : [after(VENT_PULSE_WIDTH,msec)]
  AAIR -> MAIN [order 3] : [mode ~= 7]
  MAIN -> AAI [order 3] : [mode == 3]
  AAI -> MAIN [order 3] : [mode ~= 3]
  MAIN -> AAIR [order 7] : [mode == 7]
  MAIN -> VVIR [order 8] : [mode == 8]
  VVIR -> MAIN [order 3] : [mode ~= 8]
  MAIN -> VVI [order 2] : [mode == 4]
  VVI -> MAIN [order 3] : [mode ~= 4]
  AAI -> Pacing_AAI1 [order 1] : [(ATR_CMP_DETECT==false) &&after(60000/LRL - ATR_PULSE_WIDTH-double(ARP),msec)]
  AAI -> AAI_REFRACTORY [order 2] : [ATR_CMP_DETECT == true]
  AAI_REFRACTORY -> AAI : [after(ARP,msec)]
  Pacing_AAI1 -> AAI_REFRACTORY : [ATR_CMP_DETECT == true]
  AAIR -> Pacing_AAIR [order 1] : [(ATR_CMP_DETECT==false) &&after(60000/Rate - ATR_PULSE_WIDTH - double(ARP),msec)]
  AAIR -> AAIR_REFRACTORY [order 2] : [ATR_CMP_DETECT == true]
  Pacing_AAIR -> AAIR_REFRACTORY : [ATR_CMP_DETECT == true]
  AAIR_REFRACTORY -> AAIR : [after(ARP,msec)]
  VVI -> Pacing_VVI [order 1] : [(VENT_CMP_DETECT==false) &&after(60000/LRL - VENT_PULSE_WIDTH-double(VRP),msec)]
  VVI -> VVI_REFRACTORY [order 2] : [VENT_CMP_DETECT == true]
  Pacing_VVI -> VVI_REFRACTORY : [VENT_CMP_DETECT == true]
  VVI_REFRACTORY -> VVI : [after(VRP,msec)]
  VVIR -> Pacing_VVIR [order 1] : [(VENT_CMP_DETECT==false) &&after(60000/Rate - VENT_PULSE_WIDTH-double(VRP),msec)]
  VVIR -> VVIR_REFRACTORY [order 2] : [VENT_CMP_DETECT == true]
  Pacing_VVIR -> VVIR_REFRACTORY : [VENT_CMP_DETECT == true]
  VVIR_REFRACTORY -> VVIR : [after(VRP,msec)]
  data: LRL input; VENT_Amplitude input; ATR_Amplitude input; VENT_PULSE_WIDTH input; ATR_PULSE_WIDTH input; URL input; VENTSENSITIVITY_Amplitude input; PACE_CHARGE_CTRL output; PACING_REF_PWM output; ATR_PACE_CTRL output; VENT_PACE_CTRL output; PACE_GND_CTRL output; Z_VENT_CTRL output; ATR_GND_CTRL output; VENT_GND_CTRL output; Z_ATR_CTRL output; VENT_CMP_REF_PWM output; FRONTEND_CTRL output; mode input; ATR_CMP_REF_PWM output; ATRSENSITIVITY_Amplitude input; ARP input; VRP input; Rate input; VENT_CMP_DETECT input; ATR_CMP_DETECT input

== stateflow chart Final_Simulink_Model_assignment_2/Find the desired rate for pacing1 ==
  note: Two conditions for the comparsion
  note: If our detected level is lower than or equal to the threshold
      | The desired will not increase, it will stay at LRL
  state Desired_rate_output_3
    entry:
    Desired_rate = LRL;
  state Check
    % check how the desired rate is going to change depends on activity level
  note: Loop back to the initial state and keep checking
  note: We find a higher rate when we have a larger value than the threshold
  note: Make sure the desired rate will not larger than MSR
  state Linear_increase
    entry:
    temp_rate = LRL + Response_Factor*(Activity_level-double(Activity_threshold));
  state Desired_rate_output_2
    entry:
    Desired_rate = MSR;
  state Desired_rate_output_1
    entry:
    Desired_rate = temp_rate;
  (default) -> Check
  Check -> Desired_rate_output_3 [order 2] : [Activity_level <= Activity_threshold]
  Desired_rate_output_1 -> Check : after(300,msec)
  Desired_rate_output_3 -> Check : after(300,msec)
  Check -> Linear_increase [order 1] : [Activity_level > Activity_threshold]
  Desired_rate_output_2 -> Check : after(300,msec)
  Linear_increase -> Desired_rate_output_2 [order 2] : [temp_rate >= MSR]
  Linear_increase -> Desired_rate_output_1 [order 1] : [temp_rate < MSR]
  data: Activity_level input double; LRL input; MSR input; Activity_threshold input single; Response_Factor input; Desired_rate output; temp_rate local

== stateflow chart Final_Simulink_Model_assignment_2/Find the pacing rate1 ==
  state Initial_state
    rate = LRL;
  note: Firstly define the rate to LRL
  note: If the rate is larger than our desired rate, it decreases
  note: Different increments when facing various conditions
  state Steps
    entry:
    addition = (MSR-LRL)/double(Reaction_time);
    substruction = (MSR-LRL)/double(Recovery_time);
  state Decreasing
    % using linear function to decrease
    entry:
    if(rate < MSR)
    rate = rate  - substruction;
    elseif(rate <= LRL)
    rate = LRL;
    end
  note: The rate can not be smaller than LRL
  note: Keep checking for every 300 ms
  note: Do the addition if we have a higher desired rate
  state Increasing
    % using linear function to increase
    entry:
    if(rate < MSR && rate < Desired_rate)
    rate = rate + addition;
    elseif(rate == Desired_rate)
    rate = Desired_rate;
    elseif(rate >= MSR)
    rate = MSR;
    end
  note: The rate should not exceed MSR
  (default) -> Initial_state
  Initial_state -> Steps
  Steps -> Decreasing [order 1] : after(300,msec)[rate > Desired_rate]
  Decreasing -> Steps : after(300,msec)
  Steps -> Increasing [order 2] : after(300,msec)
  Increasing -> Steps : after(300,msec)
  data: LRL input; MSR input; Desired_rate input; Reaction_time input uint8; Recovery_time input uint8; rate output; addition local; substruction local
